simulink model "SMC_rbf_intergrated_model"  (R2020b)
settings: Solver=FixedStepAuto  StartTime=0.0  StopTime=3  FixedStep=0.001  RelTol=1e-3
settings Model: Creator=Dell Precision  LastModifiedBy=Dell Precision

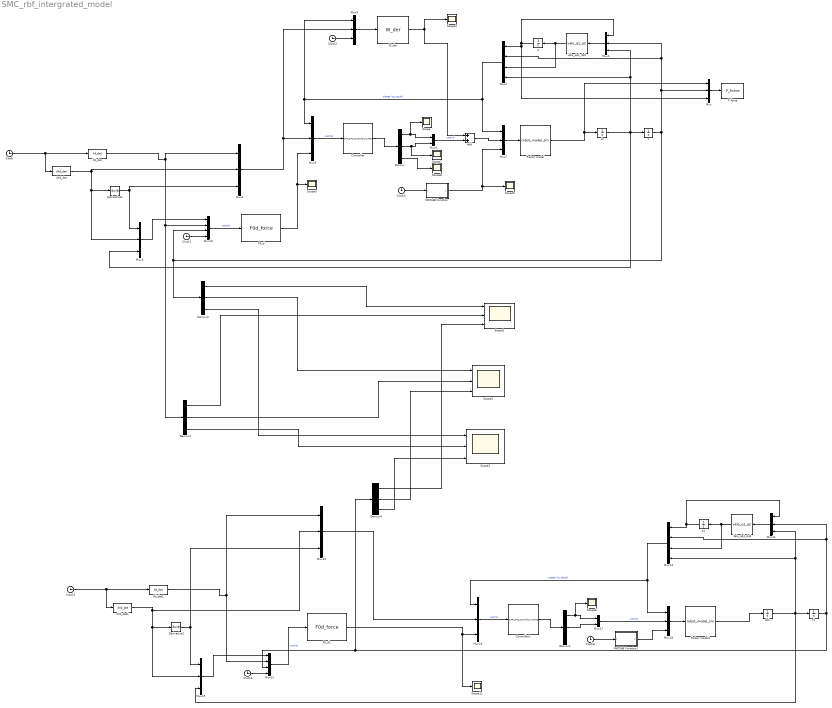
== system SMC_rbf_intergrated_model ==
  Add : Sum
  Clock{,1..6} (7 alike) : Clock
  Controller : MATLABFcn  MATLABFcn=DAR_SMC_controller_noAdap  OutputDimensions=12
  Controller1 : MATLABFcn  MATLABFcn=DAR_SMC_controller_noAdap  OutputDimensions=12
  Demux : Demux  Outputs=[3;3;6]
  Demux1 : Demux  Outputs=[3;3;6]
  Demux2 : Demux  Outputs=3
  Demux3 : Demux  Outputs=3
  Demux4 : Demux  Outputs=3
  Derivative1 : Derivative
  Derivative2 : Derivative
  F force : MATLABFcn  MATLABFcn=F_force  OutputDimensions=7
  F0_d : MATLABFcn  MATLABFcn=F0d_force  OutputDimensions=3
  F0_d1 : MATLABFcn  MATLABFcn=F0d_force  OutputDimensions=3
  MATLAB Function : MATLAB Function  TreatAsAtomicUnit=on
  MATLAB Function1 : MATLAB Function  TreatAsAtomicUnit=on
  Mux{,1,3..5,7,9,11,14..16,18} (12 alike) : Mux  Inputs=3
  Mux{2,10,12..13} (4 alike) : Mux
  Mux17 : Mux  Inputs=2
  Mux6 : Mux  Inputs=2
  Robot model : MATLABFcn  MATLABFcn=robot_model_sm  OutputDimensions=3
  Robot model1 : MATLABFcn  MATLABFcn=robot_model_sm  OutputDimensions=3
  Scope{,4..9,11} (8 alike) : Scope
  Scope1 : Scope  NumInputPorts=3
  Scope2 : Scope  NumInputPorts=3
  Scope3 : Scope  NumInputPorts=3
  Velo_dq1_dq1 : MATLABFcn  MATLABFcn=velo_q1_q2  OutputDimensions=6
  Velo_dq1_dq2 : MATLABFcn  MATLABFcn=velo_q1_q2  OutputDimensions=6
  W_der : MATLABFcn  MATLABFcn=W_der  OutputDimensions=6
  Xd_dat : MATLABFcn  MATLABFcn=Xd_dat  OutputDimensions=3
  Xd_dat1 : MATLABFcn  MATLABFcn=Xd_dat  OutputDimensions=3
  dXd_dat : MATLABFcn  MATLABFcn=dXd_dat  OutputDimensions=3
  dXd_dat1 : MATLABFcn  MATLABFcn=dXd_dat  OutputDimensions=3
  dz : Integrator  InitialCondition=[0;0;0]
  dz1 : Integrator  InitialCondition=[0;0;0]
  q : Integrator  InitialCondition=[3*pi/4;19*pi/12;5*pi/3;pi/4;5*pi/12;pi/3]  LimitOutput=on
  q1 : Integrator  InitialCondition=[3*pi/4;19*pi/12;5*pi/3;pi/4;5*pi/12;pi/3]  LimitOutput=on
  z : Integrator  InitialCondition=[0.5429;1.3999;0]  LimitOutput=on
  z1 : Integrator  InitialCondition=[0.5429;1.3999;0]  LimitOutput=on
  wires:
  Mux3/1 -> Mux5/2, Mux9/2
  dz/1 -> Mux4/3, Mux1/3, Mux2/4, z/1
  z/1 -> Mux10/3, Demux3/1, Mux1/2, Mux2/2, Mux/2
  Mux1/1 -> Velo_dq1_dq2/1
  Velo_dq1_dq2/1 -> Mux2/3, q/1
  q/1 -> Mux2/1, Mux/3, Mux1/1
  Mux/1 -> F force/1
  Clock/1 -> dXd_dat/1, Xd_dat/1
  Xd_dat/1 -> Demux2/1, Mux10/2, Mux3/1
  dXd_dat/1 -> Mux4/2, Derivative1/1, Mux3/2
  Derivative1/1 -> Mux4/1, Mux3/3
  Mux2/1 -> Mux9/1, Mux5/1, Mux7/1  "states (q,z,dq,dz)"
  Controller/1 -> Demux/1
  Demux/1 -> Scope/1, Mux6/1
  Demux/2 -> Scope7/1, Mux6/2
  Mux6/1 -> Add/2  "control"
  Mux7/1 -> Robot model/1
  Mux5/1 -> Controller/1  "control"
  Robot model/1 -> Mux/1, dz/1
  Demux3/1 -> Scope1/1
  Demux2/1 -> Scope1/2
  Demux3/2 -> Scope2/1
  Demux2/2 -> Scope2/2
  Demux3/3 -> Scope3/1
  Demux2/3 -> Scope3/2
  Mux9/1 -> W_der/1
  W_der/1 -> Scope4/1, Add/1
  Add/1 -> Mux7/2
  Clock2/1 -> Mux9/3
  Mux4/1 -> Mux10/1
  Mux10/1 -> F0_d/1  "control"
  Clock1/1 -> Mux10/4
  F0_d/1 -> Scope5/1, Mux5/3
  F0_d1/1 -> Scope11/1, Mux16/3
  Clock4/1 -> Mux12/4
  Mux12/1 -> F0_d1/1  "control"
  Mux15/1 -> Mux12/1
  Robot model1/1 -> dz1/1
  Mux16/1 -> Controller1/1  "control"
  Mux18/1 -> Robot model1/1
  Mux17/1 -> Mux18/2  "control"
  Demux1/2 -> Mux17/2
  Demux1/1 -> Mux17/1, Scope6/1
  Controller1/1 -> Demux1/1
  Mux13/1 -> Mux18/1, Mux16/1  "states (q,z,dq,dz)"
  Derivative2/1 -> Mux15/1, Mux14/3
  dXd_dat1/1 -> Derivative2/1, Mux15/2, Mux14/2
  Xd_dat1/1 -> Mux12/2, Mux14/1
  Clock3/1 -> Xd_dat1/1, dXd_dat1/1
  q1/1 -> Mux11/1, Mux13/1
  Velo_dq1_dq1/1 -> q1/1, Mux13/3
  Mux11/1 -> Velo_dq1_dq1/1
  z1/1 -> Mux13/2, Mux11/2, Demux4/1, Mux12/3
  dz1/1 -> z1/1, Mux13/4, Mux11/3, Mux15/3
  Mux14/1 -> Mux16/2
  Demux/3 -> Scope8/1
  Clock5/1 -> MATLAB Function/1(t)
  MATLAB Function/1(y) -> Scope9/1, Mux7/3
  Demux4/1 -> Scope1/3
  Demux4/2 -> Scope2/3
  Demux4/3 -> Scope3/3
  Clock6/1 -> MATLAB Function1/1(t)
  MATLAB Function1/1(y) -> Mux18/3

== matlab function SMC_rbf_intergrated_model/MATLAB Function ==
  data: t input; y output
function y = fcn(t)
y1 = 5*(2*cos(5*t) - sin(8.1*t) - sin(2.5*t)*cos(3.5*t) - sin(10.5*t+3));
 y2 = 5*(cos(8*t)^2 + sin(4.5*t-2)+3*sin(7*t)*cos(2*t)*sin(t)-cos(6.5*t));
 y3 = 0.05*(sin(4*t)-cos(3.2*t)+sin(7*t+5));
 y = [y1 y2 y3];
% y = [0 0 0];

== matlab function SMC_rbf_intergrated_model/MATLAB Function1 ==
  data: t input; y output
function y = fcn(t)
y1 = 1*(2*cos(5*t) - sin(8.1*t) - sin(2.5*t)*cos(3.5*t) - sin(10.5*t+3));
 y2 = 1*(cos(8*t)^2 + sin(4.5*t-2)+3*sin(7*t)*cos(2*t)*sin(t)-cos(6.5*t));
 y3 = 0.05*(sin(4*t)-cos(3.2*t)+sin(7*t+5));
 y = [y1 y2 y3];
